simulink model "untitled"  (R2018b)
settings: Solver=FixedStepAuto  StartTime=0.0  StopTime=500.0  FixedStep=0.01  RelTol=1e-3
values from neighbouring files (symbols this model uses):
  waveAmpTime = [t' yfin']    [makeWaveAmpTime.m]
undefined symbols (not defined in the file or in its folder): simu, waves
settings Model: Creator=glennond  LastModifiedBy=glennond

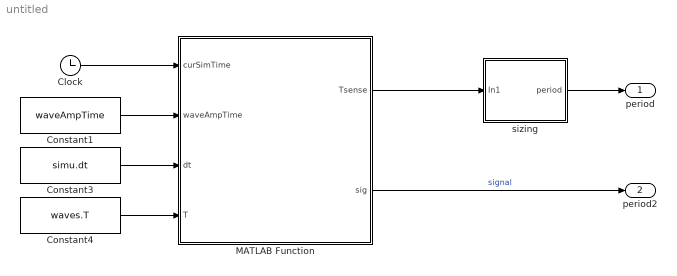
== system untitled ==
  Clock : Clock
  Constant1 : Constant  Value=waveAmpTime
  Constant3 : Constant  Value=simu.dt
  Constant4 : Constant  Value=waves.T
  MATLAB Function : MATLAB Function  TreatAsAtomicUnit=on  SystemSampleTime=0.1
  sizing : Subsystem
  period : Outport
  period2 : Outport  Port=2
  wires:
  Clock/1 -> MATLAB Function/1(curSimTime)
  Constant1/1 -> MATLAB Function/2(waveAmpTime)
  Constant3/1 -> MATLAB Function/3(dt)
  MATLAB Function/2(sig) -> period2/1  "signal"
  Constant4/1 -> MATLAB Function/4(T)
  MATLAB Function/1(Tsense) -> sizing/1(In1)
  sizing/1(period) -> period/1

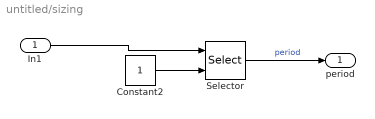
== system untitled/sizing ==
  In1 : Inport
  Constant2 : Constant
  Selector : Selector  InputPortWidth=2  IndexOptions=Index vector (port)  Indices=1  OutputSizes=1
  period : Outport
  wires:
  Constant2/1 -> Selector/2
  In1/1 -> Selector/1
  Selector/1 -> period/1  "period"

== matlab function untitled/MATLAB Function ==
  data: curSimTime input; Tsense output size=[1 2]; waveAmpTime input; dt input; sig output; T input
function [Tsense,sig] = getPeriod(curSimTime, waveAmpTime, dt, T)

% This function sort of pretends we don't know the full time series for
% wave amplitude since for control purposes, we won't. Use a rolling sample
% window of the wave height and DFT to get an approximate period for
% control purposes. This way the control can respond to a more
% "instantaneous" value for period.

if curSimTime == 0 % pre-historic...
    Tsense = T;
    sig = 0;
else
    
    t = waveAmpTime(:,1);
    eta = waveAmpTime(:,2);

    % Time series of amplitudes from simulation start to current time step
    allPastt = t(t<=curSimTime);
    allPastSamples = numel(allPastt);
    allPastEta = eta(1:allPastSamples);
    % Current Amp
    sig = allPastEta(end);

    % a 5-ish cycle sample window
    samplesPerCycle = T/dt;
    
    if curSimTime < 5*T
        windowSamples = allPastSamples; % use what we got
    else
        windowSamples = 5*samplesPerCycle;
    end

    windowPastt = allPastt(end-windowSamples+1:end);
    windowPastEta = allPastEta(end-windowSamples+1:end);

    % Sampling frequency
    fs = 1/dt;

    %Signal Length
    L = windowSamples;

    % Calculate fft
    eta_dft_mags = abs(fft(windowPastEta));

    %% Single-sided magnitude spectrum with frequency axis in Hertz
    % Each bin frequency is separated by fs/N Hertz.
    bin_vals = [0 : L-1];
    fax_Hz = bin_vals*fs/L;
    L_2 = ceil(L/2);

    freqs = fax_Hz(1:L_2);
    mags = eta_dft_mags(1:L_2);

    [~, dPd] = max(mags);
    Tsense = 1/freqs(dPd)


    if Tsense == Inf
       Tsense = T;
    end
end
end
